simulink model "Inverter2016a"  (R2016a)
settings: Solver=VariableStepAuto  SolverMode=SingleTasking  StartTime=0.0  StopTime=30e-3  FixedStep=SampleTime  MinStep=SampleTime*1e-2  RelTol=1e-3
values from neighbouring files (symbols this model uses):
  ffund = 50    [InverterMFile.m]
  ModulationIndex = 0.9    [InverterMFile.m]
  Rin = 10    [InverterMFile.m]
  Rload = Z*PF    [InverterMFile.m]
  VpulseMax = 6    [InverterMFile.m]
  VpulseMin = -3    [InverterMFile.m]
libraries: elec_lib x135, fl_lib x66, nesl_utility x65, simulink x24, powerlib_meascontrol x2
(part 4 of 4)

== system Inverter2016a/3ph- Module1/Gate Driver5 ==
  PWM : Inport
  Capacitor : elec_lib/Passive Devices/Capacitor  enable_table=0  c=142e-12 F  Cvec=[1e-05, 1e-06] F  Vvec=[0, 10] V  CV_table_symmetry=1  C_tol=5  enable_C_tol=0  tol_distribution=1  nSigma=4  r=1e-6 Ohm  g=0 1/Ohm  enable_operating_limits=0  operating_limit_action=2  max_working_voltage_range=[-25, 25] V  power_rating=1 W  enable_faults=0  fault_action=1  Cscale_faulted=100  R_faulted=1e-3 Ohm  G_faulted=0 1/Ohm  tau_fault=1e-3 s  enable_temporal_fault=0  t_fault=1 s  enable_behavioral_fault=0  max_permissible_voltage_range=[-100, 100] V  t_fail_on_voltage=1 s  i_specify=off  i_priority=None  i=0 A  i_nominal_specify=off  i_nominal_unit=A  i_nominal_value=1  v_specify=off  v_priority=None  v=0 V  v_nominal_specify=off  v_nominal_unit=V  v_nominal_value=1  vc_specify=off  vc_priority=High  vc=0 V  vc_nominal_specify=off  vc_nominal_unit=V  vc_nominal_value=1
  Current Measure : Subsystem
  Inductor : elec_lib/Passive Devices/Inductor  l=Ls H  L_tol=20  enable_L_tol=0  tol_distribution=1  nSigma=4  r=0 Ohm  g=1e-9 1/Ohm  enable_operating_limits=0  operating_limit_action=2  max_working_current=1 A  power_rating=1 W  enable_faults=0  fault_action=1  lambdaPercent=50  k_faulted=0.9999  turnsShort=0  openCct=0  groundShort=0  groundShortG=0 1/Ohm  tau_fault=1e-3 s  enable_temporal_fault=0  t_fault=1 s  enable_behavioral_fault=0  max_permissible_voltage=100 V  n_fail_on_voltage=1  max_permissible_current=1 A  t_fail_on_current=1 s  i_L_specify=off  i_L_priority=High  i_L=0 A  i_L_nominal_specify=off  i_L_nominal_unit=A  i_L_nominal_value=1
  Inductor1 : elec_lib/Passive Devices/Inductor  l=Ld H  L_tol=20  enable_L_tol=0  tol_distribution=1  nSigma=4  r=0 Ohm  g=1e-9 1/Ohm  enable_operating_limits=0  operating_limit_action=2  max_working_current=1 A  power_rating=1 W  enable_faults=0  fault_action=1  lambdaPercent=50  k_faulted=0.9999  turnsShort=0  openCct=0  groundShort=0  groundShortG=0 1/Ohm  tau_fault=1e-3 s  enable_temporal_fault=0  t_fault=1 s  enable_behavioral_fault=0  max_permissible_voltage=100 V  n_fail_on_voltage=1  max_permissible_current=1 A  t_fail_on_current=1 s  i_L_specify=off  i_L_priority=High  i_L=0 A  i_L_nominal_specify=off  i_L_nominal_unit=A  i_L_nominal_value=1
  Rate Limiter2 : Subsystem
  Simulink-PS Converter : nesl_utility/Simulink-PS Converter  PhysicalDomain=network_engine_domain  SubClassName=ps_input  LeftPortType=input  RightPortType=output  PseudoPeriodic=off  Frequencies=[]  NoiseDistribution=none  NoiseParameters=[]  Unit=1  AffineConversion=off  FilteringAndDerivatives=zero  SimscapeFilterOrder=1  InputFilterTimeConstant=0.001  UdotUserProvided=1
  Switch6 : fl_lib/Electrical/Electrical Elements/Switch  R_closed=0.05 Ohm  G_open=1e-8 1/Ohm  Threshold=1.7  i_specify=off  i_priority=None  i=0 A  i_nominal_specify=off  i_nominal_unit=A  i_nominal_value=1  v_specify=off  v_priority=None  v=0 V  v_nominal_specify=off  v_nominal_unit=V  v_nominal_value=1
  Voltage Measure3 : Subsystem
  Drain : PMIOPort  Side=Left
  Source : PMIOPort  Port=2  Side=Right
  Volt : Outport
  Curr : Outport  Port=2
  wires:
  Current Measure/1(Data) -> Curr/1
  Voltage Measure3/1(Data) -> Volt/1
  Rate Limiter2/1(Outp) -> Simulink-PS Converter/1
  PWM/1 -> Rate Limiter2/1(Inp)
  connections:
  Current Measure/RConn1 -- Inductor1/RConn1
  Inductor/RConn1 -- Source/RConn1
  Current Measure/LConn1 -- Drain/RConn1
  Inductor1/LConn1 -- Capacitor/LConn1 -- Switch6/LConn1 -- Voltage Measure3/RConn1
  Capacitor/RConn1 -- Voltage Measure3/RConn2 -- Switch6/RConn2 -- Inductor/LConn1
  Switch6/RConn1 -- Simulink-PS Converter/RConn1

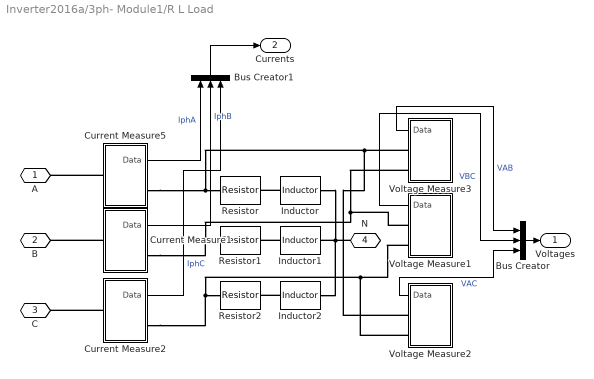
== system Inverter2016a/3ph- Module1/R L Load ==
  Bus Creator : BusCreator  Inputs=3
  Bus Creator1 : BusCreator  Inputs=3
  Current Measure1 : Subsystem
  Current Measure2 : Subsystem
  Current Measure5 : Subsystem
  Inductor : elec_lib/Passive Devices/Inductor  l=Lload H  L_tol=20  enable_L_tol=0  tol_distribution=1  nSigma=4  r=0 Ohm  g=1e-9 1/Ohm  enable_operating_limits=0  operating_limit_action=2  max_working_current=1 A  power_rating=1 W  enable_faults=0  fault_action=1  lambdaPercent=50  k_faulted=0.9999  turnsShort=0  openCct=0  groundShort=0  groundShortG=0 1/Ohm  tau_fault=0.001 s  enable_temporal_fault=0  t_fault=1 s  enable_behavioral_fault=0  max_permissible_voltage=100 V  n_fail_on_voltage=1  max_permissible_current=1 A  t_fail_on_current=1 s  i_L_specify=on  i_L_priority=High  i_L=LoadA A  i_L_nominal_specify=off  i_L_nominal_unit=A  i_L_nominal_value=1
  Inductor1 : elec_lib/Passive Devices/Inductor  l=Lload H  L_tol=20  enable_L_tol=0  tol_distribution=1  nSigma=4  r=0 Ohm  g=1e-9 1/Ohm  enable_operating_limits=0  operating_limit_action=2  max_working_current=1 A  power_rating=1 W  enable_faults=0  fault_action=1  lambdaPercent=50  k_faulted=0.9999  turnsShort=0  openCct=0  groundShort=0  groundShortG=0 1/Ohm  tau_fault=0.001 s  enable_temporal_fault=0  t_fault=1 s  enable_behavioral_fault=0  max_permissible_voltage=100 V  n_fail_on_voltage=1  max_permissible_current=1 A  t_fail_on_current=1 s  i_L_specify=on  i_L_priority=High  i_L=LoadB A  i_L_nominal_specify=off  i_L_nominal_unit=A  i_L_nominal_value=1
  Inductor2 : elec_lib/Passive Devices/Inductor  l=Lload H  L_tol=20  enable_L_tol=0  tol_distribution=1  nSigma=4  r=0 Ohm  g=1e-9 1/Ohm  enable_operating_limits=0  operating_limit_action=2  max_working_current=1 A  power_rating=1 W  enable_faults=0  fault_action=1  lambdaPercent=50  k_faulted=0.9999  turnsShort=0  openCct=0  groundShort=0  groundShortG=0 1/Ohm  tau_fault=0.001 s  enable_temporal_fault=0  t_fault=1 s  enable_behavioral_fault=0  max_permissible_voltage=100 V  n_fail_on_voltage=1  max_permissible_current=1 A  t_fail_on_current=1 s  i_L_specify=on  i_L_priority=High  i_L=LoadC A  i_L_nominal_specify=off  i_L_nominal_unit=A  i_L_nominal_value=1
  Resistor : elec_lib/Passive Devices/Resistor  R=Rload Ohm  R_tol=5  enable_R_tol=0  tol_distribution=1  nSigma=4  enable_operating_limits=0  operating_limit_action=2  max_working_voltage=100 V  power_rating=1 W  enable_faults=0  fault_action=1  R_faulted=Inf Ohm  enable_temporal_fault=0  t_fault=1 s  enable_behavioral_fault=0  max_permissible_current=1 A  t_fail_on_current=1 s  noise_mode=0  sample_time=0.001 s  repeatability=1  auto_seed=851356125  user_seed=0  Tdevice=25 degC  alpha=3.93e-3 1/K  Tmeas=25 degC  thermal_mass=100 J/K  power_derating_T1=70 degC  power_derating_T2=155 degC  operating_temperature_range_vec=[-50, 150] degC  temperature_specify=off  temperature_priority=High  temperature=298.15 K  temperature_nominal_specify=off  temperature_nominal_unit=K  temperature_nominal_value=1
  Resistor1 : elec_lib/Passive Devices/Resistor  R=Rload Ohm  R_tol=5  enable_R_tol=0  tol_distribution=1  nSigma=4  enable_operating_limits=0  operating_limit_action=2  max_working_voltage=100 V  power_rating=1 W  enable_faults=0  fault_action=1  R_faulted=Inf Ohm  enable_temporal_fault=0  t_fault=1 s  enable_behavioral_fault=0  max_permissible_current=1 A  t_fail_on_current=1 s  noise_mode=0  sample_time=0.001 s  repeatability=1  auto_seed=837825856  user_seed=0  Tdevice=25 degC  alpha=3.93e-3 1/K  Tmeas=25 degC  thermal_mass=100 J/K  power_derating_T1=70 degC  power_derating_T2=155 degC  operating_temperature_range_vec=[-50, 150] degC  temperature_specify=off  temperature_priority=High  temperature=298.15 K  temperature_nominal_specify=off  temperature_nominal_unit=K  temperature_nominal_value=1
  Resistor2 : elec_lib/Passive Devices/Resistor  R=Rload Ohm  R_tol=5  enable_R_tol=0  tol_distribution=1  nSigma=4  enable_operating_limits=0  operating_limit_action=2  max_working_voltage=100 V  power_rating=1 W  enable_faults=0  fault_action=1  R_faulted=Inf Ohm  enable_temporal_fault=0  t_fault=1 s  enable_behavioral_fault=0  max_permissible_current=1 A  t_fail_on_current=1 s  noise_mode=0  sample_time=0.001 s  repeatability=1  auto_seed=1403765601  user_seed=0  Tdevice=25 degC  alpha=3.93e-3 1/K  Tmeas=25 degC  thermal_mass=100 J/K  power_derating_T1=70 degC  power_derating_T2=155 degC  operating_temperature_range_vec=[-50, 150] degC  temperature_specify=off  temperature_priority=High  temperature=298.15 K  temperature_nominal_specify=off  temperature_nominal_unit=K  temperature_nominal_value=1
  Voltage Measure1 : Subsystem
  Voltage Measure2 : Subsystem
  Voltage Measure3 : Subsystem
  A : PMIOPort  Side=Left
  B : PMIOPort  Port=2  Side=Left
  C : PMIOPort  Port=3  Side=Left
  N : PMIOPort  Port=4  Side=Right
  Voltages : Outport
  Currents : Outport  Port=2
  wires:
  Bus Creator1/1 -> Currents/1
  Bus Creator/1 -> Voltages/1
  Current Measure2/1(Data) -> Bus Creator1/3  "IphC"
  Current Measure1/1(Data) -> Bus Creator1/2  "IphB"
  Current Measure5/1(Data) -> Bus Creator1/1  "IphA"
  Voltage Measure2/1(Data) -> Bus Creator/3  "VAC"
  Voltage Measure1/1(Data) -> Bus Creator/2  "VBC"
  Voltage Measure3/1(Data) -> Bus Creator/1  "VAB"
  connections:
  Current Measure2/LConn1 -- C/RConn1
  Current Measure1/LConn1 -- B/RConn1
  Current Measure5/LConn1 -- A/RConn1
  Resistor2/LConn1 -- Voltage Measure1/RConn2 -- Voltage Measure2/RConn2 -- Current Measure2/RConn1
  Resistor/LConn1 -- Voltage Measure3/RConn1 -- Voltage Measure2/RConn1 -- Current Measure5/RConn1
  Resistor1/LConn1 -- Voltage Measure3/RConn2 -- Voltage Measure1/RConn1 -- Current Measure1/RConn1
  Inductor1/LConn1 -- Resistor1/RConn1
  Inductor2/LConn1 -- Resistor2/RConn1
  N/RConn1 -- Inductor1/RConn1 -- Inductor2/RConn1 -- Inductor/RConn1
  Inductor/LConn1 -- Resistor/RConn1

== system Inverter2016a/3ph- Module1/Voltage Measure1 ==
  PS-Simulink Converter2 : nesl_utility/PS-Simulink Converter  PhysicalDomain=network_engine_domain  SubClassName=ps_output  LeftPortType=input  RightPortType=output  PseudoPeriodic=off  Frequencies=[]  Unit=1  AffineConversion=off
  Voltage Sensor3 : fl_lib/Electrical/Electrical Sensors/Voltage Sensor
  V+ : PMIOPort  Side=Right
  V- : PMIOPort  Port=2  Side=Right
  Data : Outport
  wires:
  PS-Simulink Converter2/1 -> Data/1
  connections:
  PS-Simulink Converter2/LConn1 -- Voltage Sensor3/RConn1
  Voltage Sensor3/RConn2 -- V-/RConn1
  Voltage Sensor3/LConn1 -- V+/RConn1

== system Inverter2016a/3ph- Module1/Voltage Measure2 ==
  PS-Simulink Converter2 : nesl_utility/PS-Simulink Converter  PhysicalDomain=network_engine_domain  SubClassName=ps_output  LeftPortType=input  RightPortType=output  PseudoPeriodic=off  Frequencies=[]  Unit=1  AffineConversion=off
  Voltage Sensor3 : fl_lib/Electrical/Electrical Sensors/Voltage Sensor
  V+ : PMIOPort  Side=Right
  V- : PMIOPort  Port=2  Side=Right
  Data : Outport
  wires:
  PS-Simulink Converter2/1 -> Data/1
  connections:
  PS-Simulink Converter2/LConn1 -- Voltage Sensor3/RConn1
  Voltage Sensor3/RConn2 -- V-/RConn1
  Voltage Sensor3/LConn1 -- V+/RConn1

== system Inverter2016a/3ph- Module1/Voltage Measure3 ==
  PS-Simulink Converter2 : nesl_utility/PS-Simulink Converter  PhysicalDomain=network_engine_domain  SubClassName=ps_output  LeftPortType=input  RightPortType=output  PseudoPeriodic=off  Frequencies=[]  Unit=1  AffineConversion=off
  Voltage Sensor3 : fl_lib/Electrical/Electrical Sensors/Voltage Sensor
  V+ : PMIOPort  Side=Right
  V- : PMIOPort  Port=2  Side=Right
  Data : Outport
  wires:
  PS-Simulink Converter2/1 -> Data/1
  connections:
  PS-Simulink Converter2/LConn1 -- Voltage Sensor3/RConn1
  Voltage Sensor3/RConn2 -- V-/RConn1
  Voltage Sensor3/LConn1 -- V+/RConn1

== system Inverter2016a/3ph- Module1/Voltage Measure4 ==
  PS-Simulink Converter2 : nesl_utility/PS-Simulink Converter  PhysicalDomain=network_engine_domain  SubClassName=ps_output  LeftPortType=input  RightPortType=output  PseudoPeriodic=off  Frequencies=[]  Unit=1  AffineConversion=off
  Voltage Sensor3 : fl_lib/Electrical/Electrical Sensors/Voltage Sensor
  V+ : PMIOPort  Side=Right
  V- : PMIOPort  Port=2  Side=Right
  Data : Outport
  wires:
  PS-Simulink Converter2/1 -> Data/1
  connections:
  Voltage Sensor3/LConn1 -- V+/RConn1
  Voltage Sensor3/RConn2 -- V-/RConn1
  PS-Simulink Converter2/LConn1 -- Voltage Sensor3/RConn1

== system Inverter2016a/3ph- Module/Gate Driver/Current Measure ==
  Current Sensor1 : fl_lib/Electrical/Electrical Sensors/Current Sensor
  PS-Simulink Converter4 : nesl_utility/PS-Simulink Converter  PhysicalDomain=network_engine_domain  SubClassName=ps_output  LeftPortType=input  RightPortType=output  PseudoPeriodic=off  Frequencies=[]  Unit=1  AffineConversion=off
  I+ : PMIOPort  Side=Left
  I- : PMIOPort  Port=2  Side=Right
  Data : Outport
  wires:
  PS-Simulink Converter4/1 -> Data/1
  connections:
  Current Sensor1/RConn2 -- I-/RConn1
  PS-Simulink Converter4/LConn1 -- Current Sensor1/RConn1
  Current Sensor1/LConn1 -- I+/RConn1

== system Inverter2016a/3ph- Module/Gate Driver/Rate Limiter2 ==
  Inp : Inport
  Constant2 : Constant  Value=(VpulseMax - VpulseMin)/1e-9
  Constant3 : Constant  Value=(VpulseMin - VpulseMax)/1e-9
  Rate Limiter Dynamic : simulink/Discontinuities/Rate Limiter Dynamic
  Outp : Outport
  wires:
  Constant3/1 -> Rate Limiter Dynamic/3
  Constant2/1 -> Rate Limiter Dynamic/1
  Inp/1 -> Rate Limiter Dynamic/2
  Rate Limiter Dynamic/1 -> Outp/1

== system Inverter2016a/3ph- Module/Gate Driver/Voltage Measure3 ==
  PS-Simulink Converter2 : nesl_utility/PS-Simulink Converter  PhysicalDomain=network_engine_domain  SubClassName=ps_output  LeftPortType=input  RightPortType=output  PseudoPeriodic=off  Frequencies=[]  Unit=1  AffineConversion=off
  Voltage Sensor3 : fl_lib/Electrical/Electrical Sensors/Voltage Sensor
  V+ : PMIOPort  Side=Right
  V- : PMIOPort  Port=2  Side=Right
  Data : Outport
  wires:
  PS-Simulink Converter2/1 -> Data/1
  connections:
  Voltage Sensor3/LConn1 -- V+/RConn1
  Voltage Sensor3/RConn2 -- V-/RConn1
  PS-Simulink Converter2/LConn1 -- Voltage Sensor3/RConn1

== system Inverter2016a/3ph- Module/Gate Driver1/Current Measure ==
  Current Sensor1 : fl_lib/Electrical/Electrical Sensors/Current Sensor
  PS-Simulink Converter4 : nesl_utility/PS-Simulink Converter  PhysicalDomain=network_engine_domain  SubClassName=ps_output  LeftPortType=input  RightPortType=output  PseudoPeriodic=off  Frequencies=[]  Unit=1  AffineConversion=off
  I+ : PMIOPort  Side=Left
  I- : PMIOPort  Port=2  Side=Right
  Data : Outport
  wires:
  PS-Simulink Converter4/1 -> Data/1
  connections:
  Current Sensor1/RConn2 -- I-/RConn1
  PS-Simulink Converter4/LConn1 -- Current Sensor1/RConn1
  Current Sensor1/LConn1 -- I+/RConn1

== system Inverter2016a/3ph- Module/Gate Driver1/Rate Limiter2 ==
  Inp : Inport
  Constant2 : Constant  Value=(VpulseMax - VpulseMin)/1e-9
  Constant3 : Constant  Value=(VpulseMin - VpulseMax)/1e-9
  Rate Limiter Dynamic : simulink/Discontinuities/Rate Limiter Dynamic
  Outp : Outport
  wires:
  Constant3/1 -> Rate Limiter Dynamic/3
  Constant2/1 -> Rate Limiter Dynamic/1
  Inp/1 -> Rate Limiter Dynamic/2
  Rate Limiter Dynamic/1 -> Outp/1

== system Inverter2016a/3ph- Module/Gate Driver1/Voltage Measure3 ==
  PS-Simulink Converter2 : nesl_utility/PS-Simulink Converter  PhysicalDomain=network_engine_domain  SubClassName=ps_output  LeftPortType=input  RightPortType=output  PseudoPeriodic=off  Frequencies=[]  Unit=1  AffineConversion=off
  Voltage Sensor3 : fl_lib/Electrical/Electrical Sensors/Voltage Sensor
  V+ : PMIOPort  Side=Right
  V- : PMIOPort  Port=2  Side=Right
  Data : Outport
  wires:
  PS-Simulink Converter2/1 -> Data/1
  connections:
  Voltage Sensor3/LConn1 -- V+/RConn1
  Voltage Sensor3/RConn2 -- V-/RConn1
  PS-Simulink Converter2/LConn1 -- Voltage Sensor3/RConn1

== system Inverter2016a/3ph- Module/Gate Driver2/Current Measure ==
  Current Sensor1 : fl_lib/Electrical/Electrical Sensors/Current Sensor
  PS-Simulink Converter4 : nesl_utility/PS-Simulink Converter  PhysicalDomain=network_engine_domain  SubClassName=ps_output  LeftPortType=input  RightPortType=output  PseudoPeriodic=off  Frequencies=[]  Unit=1  AffineConversion=off
  I+ : PMIOPort  Side=Left
  I- : PMIOPort  Port=2  Side=Right
  Data : Outport
  wires:
  PS-Simulink Converter4/1 -> Data/1
  connections:
  Current Sensor1/RConn2 -- I-/RConn1
  PS-Simulink Converter4/LConn1 -- Current Sensor1/RConn1
  Current Sensor1/LConn1 -- I+/RConn1

== system Inverter2016a/3ph- Module/Gate Driver2/Rate Limiter2 ==
  Inp : Inport
  Constant2 : Constant  Value=(VpulseMax - VpulseMin)/1e-9
  Constant3 : Constant  Value=(VpulseMin - VpulseMax)/1e-9
  Rate Limiter Dynamic : simulink/Discontinuities/Rate Limiter Dynamic
  Outp : Outport
  wires:
  Constant3/1 -> Rate Limiter Dynamic/3
  Constant2/1 -> Rate Limiter Dynamic/1
  Inp/1 -> Rate Limiter Dynamic/2
  Rate Limiter Dynamic/1 -> Outp/1

== system Inverter2016a/3ph- Module/Gate Driver2/Voltage Measure3 ==
  PS-Simulink Converter2 : nesl_utility/PS-Simulink Converter  PhysicalDomain=network_engine_domain  SubClassName=ps_output  LeftPortType=input  RightPortType=output  PseudoPeriodic=off  Frequencies=[]  Unit=1  AffineConversion=off
  Voltage Sensor3 : fl_lib/Electrical/Electrical Sensors/Voltage Sensor
  V+ : PMIOPort  Side=Right
  V- : PMIOPort  Port=2  Side=Right
  Data : Outport
  wires:
  PS-Simulink Converter2/1 -> Data/1
  connections:
  Voltage Sensor3/LConn1 -- V+/RConn1
  Voltage Sensor3/RConn2 -- V-/RConn1
  PS-Simulink Converter2/LConn1 -- Voltage Sensor3/RConn1

== system Inverter2016a/3ph- Module/Gate Driver3/Current Measure ==
  Current Sensor1 : fl_lib/Electrical/Electrical Sensors/Current Sensor
  PS-Simulink Converter4 : nesl_utility/PS-Simulink Converter  PhysicalDomain=network_engine_domain  SubClassName=ps_output  LeftPortType=input  RightPortType=output  PseudoPeriodic=off  Frequencies=[]  Unit=1  AffineConversion=off
  I+ : PMIOPort  Side=Left
  I- : PMIOPort  Port=2  Side=Right
  Data : Outport
  wires:
  PS-Simulink Converter4/1 -> Data/1
  connections:
  Current Sensor1/RConn2 -- I-/RConn1
  PS-Simulink Converter4/LConn1 -- Current Sensor1/RConn1
  Current Sensor1/LConn1 -- I+/RConn1

== system Inverter2016a/3ph- Module/Gate Driver3/Rate Limiter2 ==
  Inp : Inport
  Constant2 : Constant  Value=(VpulseMax - VpulseMin)/1e-9
  Constant3 : Constant  Value=(VpulseMin - VpulseMax)/1e-9
  Rate Limiter Dynamic : simulink/Discontinuities/Rate Limiter Dynamic
  Outp : Outport
  wires:
  Constant3/1 -> Rate Limiter Dynamic/3
  Constant2/1 -> Rate Limiter Dynamic/1
  Inp/1 -> Rate Limiter Dynamic/2
  Rate Limiter Dynamic/1 -> Outp/1

== system Inverter2016a/3ph- Module/Gate Driver3/Voltage Measure3 ==
  PS-Simulink Converter2 : nesl_utility/PS-Simulink Converter  PhysicalDomain=network_engine_domain  SubClassName=ps_output  LeftPortType=input  RightPortType=output  PseudoPeriodic=off  Frequencies=[]  Unit=1  AffineConversion=off
  Voltage Sensor3 : fl_lib/Electrical/Electrical Sensors/Voltage Sensor
  V+ : PMIOPort  Side=Right
  V- : PMIOPort  Port=2  Side=Right
  Data : Outport
  wires:
  PS-Simulink Converter2/1 -> Data/1
  connections:
  Voltage Sensor3/LConn1 -- V+/RConn1
  Voltage Sensor3/RConn2 -- V-/RConn1
  PS-Simulink Converter2/LConn1 -- Voltage Sensor3/RConn1

== system Inverter2016a/3ph- Module/Gate Driver4/Current Measure ==
  Current Sensor1 : fl_lib/Electrical/Electrical Sensors/Current Sensor
  PS-Simulink Converter4 : nesl_utility/PS-Simulink Converter  PhysicalDomain=network_engine_domain  SubClassName=ps_output  LeftPortType=input  RightPortType=output  PseudoPeriodic=off  Frequencies=[]  Unit=1  AffineConversion=off
  I+ : PMIOPort  Side=Left
  I- : PMIOPort  Port=2  Side=Right
  Data : Outport
  wires:
  PS-Simulink Converter4/1 -> Data/1
  connections:
  Current Sensor1/RConn2 -- I-/RConn1
  PS-Simulink Converter4/LConn1 -- Current Sensor1/RConn1
  Current Sensor1/LConn1 -- I+/RConn1

== system Inverter2016a/3ph- Module/Gate Driver4/Rate Limiter2 ==
  Inp : Inport
  Constant2 : Constant  Value=(VpulseMax - VpulseMin)/1e-9
  Constant3 : Constant  Value=(VpulseMin - VpulseMax)/1e-9
  Rate Limiter Dynamic : simulink/Discontinuities/Rate Limiter Dynamic
  Outp : Outport
  wires:
  Constant3/1 -> Rate Limiter Dynamic/3
  Constant2/1 -> Rate Limiter Dynamic/1
  Inp/1 -> Rate Limiter Dynamic/2
  Rate Limiter Dynamic/1 -> Outp/1

== system Inverter2016a/3ph- Module/Gate Driver4/Voltage Measure3 ==
  PS-Simulink Converter2 : nesl_utility/PS-Simulink Converter  PhysicalDomain=network_engine_domain  SubClassName=ps_output  LeftPortType=input  RightPortType=output  PseudoPeriodic=off  Frequencies=[]  Unit=1  AffineConversion=off
  Voltage Sensor3 : fl_lib/Electrical/Electrical Sensors/Voltage Sensor
  V+ : PMIOPort  Side=Right
  V- : PMIOPort  Port=2  Side=Right
  Data : Outport
  wires:
  PS-Simulink Converter2/1 -> Data/1
  connections:
  Voltage Sensor3/LConn1 -- V+/RConn1
  Voltage Sensor3/RConn2 -- V-/RConn1
  PS-Simulink Converter2/LConn1 -- Voltage Sensor3/RConn1

== system Inverter2016a/3ph- Module/Gate Driver5/Current Measure ==
  Current Sensor1 : fl_lib/Electrical/Electrical Sensors/Current Sensor
  PS-Simulink Converter4 : nesl_utility/PS-Simulink Converter  PhysicalDomain=network_engine_domain  SubClassName=ps_output  LeftPortType=input  RightPortType=output  PseudoPeriodic=off  Frequencies=[]  Unit=1  AffineConversion=off
  I+ : PMIOPort  Side=Left
  I- : PMIOPort  Port=2  Side=Right
  Data : Outport
  wires:
  PS-Simulink Converter4/1 -> Data/1
  connections:
  Current Sensor1/RConn2 -- I-/RConn1
  PS-Simulink Converter4/LConn1 -- Current Sensor1/RConn1
  Current Sensor1/LConn1 -- I+/RConn1

== system Inverter2016a/3ph- Module/Gate Driver5/Rate Limiter2 ==
  Inp : Inport
  Constant2 : Constant  Value=(VpulseMax - VpulseMin)/1e-9
  Constant3 : Constant  Value=(VpulseMin - VpulseMax)/1e-9
  Rate Limiter Dynamic : simulink/Discontinuities/Rate Limiter Dynamic
  Outp : Outport
  wires:
  Constant3/1 -> Rate Limiter Dynamic/3
  Constant2/1 -> Rate Limiter Dynamic/1
  Inp/1 -> Rate Limiter Dynamic/2
  Rate Limiter Dynamic/1 -> Outp/1

== system Inverter2016a/3ph- Module/Gate Driver5/Voltage Measure3 ==
  PS-Simulink Converter2 : nesl_utility/PS-Simulink Converter  PhysicalDomain=network_engine_domain  SubClassName=ps_output  LeftPortType=input  RightPortType=output  PseudoPeriodic=off  Frequencies=[]  Unit=1  AffineConversion=off
  Voltage Sensor3 : fl_lib/Electrical/Electrical Sensors/Voltage Sensor
  V+ : PMIOPort  Side=Right
  V- : PMIOPort  Port=2  Side=Right
  Data : Outport
  wires:
  PS-Simulink Converter2/1 -> Data/1
  connections:
  Voltage Sensor3/LConn1 -- V+/RConn1
  Voltage Sensor3/RConn2 -- V-/RConn1
  PS-Simulink Converter2/LConn1 -- Voltage Sensor3/RConn1

== system Inverter2016a/3ph- Module/R L Load/Current Measure1 ==
  Current Sensor1 : fl_lib/Electrical/Electrical Sensors/Current Sensor
  PS-Simulink Converter4 : nesl_utility/PS-Simulink Converter  PhysicalDomain=network_engine_domain  SubClassName=ps_output  LeftPortType=input  RightPortType=output  PseudoPeriodic=off  Frequencies=[]  Unit=1  AffineConversion=off
  I+ : PMIOPort  Side=Left
  I- : PMIOPort  Port=2  Side=Right
  Data : Outport
  wires:
  PS-Simulink Converter4/1 -> Data/1
  connections:
  Current Sensor1/LConn1 -- I+/RConn1
  PS-Simulink Converter4/LConn1 -- Current Sensor1/RConn1
  Current Sensor1/RConn2 -- I-/RConn1

== system Inverter2016a/3ph- Module/R L Load/Current Measure2 ==
  Current Sensor1 : fl_lib/Electrical/Electrical Sensors/Current Sensor
  PS-Simulink Converter4 : nesl_utility/PS-Simulink Converter  PhysicalDomain=network_engine_domain  SubClassName=ps_output  LeftPortType=input  RightPortType=output  PseudoPeriodic=off  Frequencies=[]  Unit=1  AffineConversion=off
  I+ : PMIOPort  Side=Left
  I- : PMIOPort  Port=2  Side=Right
  Data : Outport
  wires:
  PS-Simulink Converter4/1 -> Data/1
  connections:
  Current Sensor1/RConn2 -- I-/RConn1
  PS-Simulink Converter4/LConn1 -- Current Sensor1/RConn1
  Current Sensor1/LConn1 -- I+/RConn1

== system Inverter2016a/3ph- Module/R L Load/Current Measure5 ==
  Current Sensor1 : fl_lib/Electrical/Electrical Sensors/Current Sensor
  PS-Simulink Converter4 : nesl_utility/PS-Simulink Converter  PhysicalDomain=network_engine_domain  SubClassName=ps_output  LeftPortType=input  RightPortType=output  PseudoPeriodic=off  Frequencies=[]  Unit=1  AffineConversion=off
  I+ : PMIOPort  Side=Left
  I- : PMIOPort  Port=2  Side=Right
  Data : Outport
  wires:
  PS-Simulink Converter4/1 -> Data/1
  connections:
  Current Sensor1/RConn2 -- I-/RConn1
  PS-Simulink Converter4/LConn1 -- Current Sensor1/RConn1
  Current Sensor1/LConn1 -- I+/RConn1

== system Inverter2016a/3ph- Module/R L Load/Voltage Measure1 ==
  PS-Simulink Converter2 : nesl_utility/PS-Simulink Converter  PhysicalDomain=network_engine_domain  SubClassName=ps_output  LeftPortType=input  RightPortType=output  PseudoPeriodic=off  Frequencies=[]  Unit=1  AffineConversion=off
  Voltage Sensor3 : fl_lib/Electrical/Electrical Sensors/Voltage Sensor
  V+ : PMIOPort  Side=Right
  V- : PMIOPort  Port=2  Side=Right
  Data : Outport
  wires:
  PS-Simulink Converter2/1 -> Data/1
  connections:
  PS-Simulink Converter2/LConn1 -- Voltage Sensor3/RConn1
  Voltage Sensor3/RConn2 -- V-/RConn1
  Voltage Sensor3/LConn1 -- V+/RConn1

== system Inverter2016a/3ph- Module/R L Load/Voltage Measure2 ==
  PS-Simulink Converter2 : nesl_utility/PS-Simulink Converter  PhysicalDomain=network_engine_domain  SubClassName=ps_output  LeftPortType=input  RightPortType=output  PseudoPeriodic=off  Frequencies=[]  Unit=1  AffineConversion=off
  Voltage Sensor3 : fl_lib/Electrical/Electrical Sensors/Voltage Sensor
  V+ : PMIOPort  Side=Right
  V- : PMIOPort  Port=2  Side=Right
  Data : Outport
  wires:
  PS-Simulink Converter2/1 -> Data/1
  connections:
  Voltage Sensor3/LConn1 -- V+/RConn1
  Voltage Sensor3/RConn2 -- V-/RConn1
  PS-Simulink Converter2/LConn1 -- Voltage Sensor3/RConn1

== system Inverter2016a/3ph- Module/R L Load/Voltage Measure3 ==
  PS-Simulink Converter2 : nesl_utility/PS-Simulink Converter  PhysicalDomain=network_engine_domain  SubClassName=ps_output  LeftPortType=input  RightPortType=output  PseudoPeriodic=off  Frequencies=[]  Unit=1  AffineConversion=off
  Voltage Sensor3 : fl_lib/Electrical/Electrical Sensors/Voltage Sensor
  V+ : PMIOPort  Side=Right
  V- : PMIOPort  Port=2  Side=Right
  Data : Outport
  wires:
  PS-Simulink Converter2/1 -> Data/1
  connections:
  Voltage Sensor3/LConn1 -- V+/RConn1
  Voltage Sensor3/RConn2 -- V-/RConn1
  PS-Simulink Converter2/LConn1 -- Voltage Sensor3/RConn1

== system Inverter2016a/3ph- Module1/Gate Driver/Current Measure ==
  Current Sensor1 : fl_lib/Electrical/Electrical Sensors/Current Sensor
  PS-Simulink Converter4 : nesl_utility/PS-Simulink Converter  PhysicalDomain=network_engine_domain  SubClassName=ps_output  LeftPortType=input  RightPortType=output  PseudoPeriodic=off  Frequencies=[]  Unit=1  AffineConversion=off
  I+ : PMIOPort  Side=Left
  I- : PMIOPort  Port=2  Side=Right
  Data : Outport
  wires:
  PS-Simulink Converter4/1 -> Data/1
  connections:
  Current Sensor1/LConn1 -- I+/RConn1
  PS-Simulink Converter4/LConn1 -- Current Sensor1/RConn1
  Current Sensor1/RConn2 -- I-/RConn1

== system Inverter2016a/3ph- Module1/Gate Driver/Rate Limiter2 ==
  Inp : Inport
  Constant2 : Constant  Value=(VpulseMax - VpulseMin)/1e-9
  Constant3 : Constant  Value=(VpulseMin - VpulseMax)/1e-9
  Rate Limiter Dynamic : simulink/Discontinuities/Rate Limiter Dynamic
  Outp : Outport
  wires:
  Rate Limiter Dynamic/1 -> Outp/1
  Inp/1 -> Rate Limiter Dynamic/2
  Constant2/1 -> Rate Limiter Dynamic/1
  Constant3/1 -> Rate Limiter Dynamic/3

== system Inverter2016a/3ph- Module1/Gate Driver/Voltage Measure3 ==
  PS-Simulink Converter2 : nesl_utility/PS-Simulink Converter  PhysicalDomain=network_engine_domain  SubClassName=ps_output  LeftPortType=input  RightPortType=output  PseudoPeriodic=off  Frequencies=[]  Unit=1  AffineConversion=off
  Voltage Sensor3 : fl_lib/Electrical/Electrical Sensors/Voltage Sensor
  V+ : PMIOPort  Side=Right
  V- : PMIOPort  Port=2  Side=Right
  Data : Outport
  wires:
  PS-Simulink Converter2/1 -> Data/1
  connections:
  PS-Simulink Converter2/LConn1 -- Voltage Sensor3/RConn1
  Voltage Sensor3/RConn2 -- V-/RConn1
  Voltage Sensor3/LConn1 -- V+/RConn1

== system Inverter2016a/3ph- Module1/Gate Driver1/Current Measure ==
  Current Sensor1 : fl_lib/Electrical/Electrical Sensors/Current Sensor
  PS-Simulink Converter4 : nesl_utility/PS-Simulink Converter  PhysicalDomain=network_engine_domain  SubClassName=ps_output  LeftPortType=input  RightPortType=output  PseudoPeriodic=off  Frequencies=[]  Unit=1  AffineConversion=off
  I+ : PMIOPort  Side=Left
  I- : PMIOPort  Port=2  Side=Right
  Data : Outport
  wires:
  PS-Simulink Converter4/1 -> Data/1
  connections:
  Current Sensor1/LConn1 -- I+/RConn1
  PS-Simulink Converter4/LConn1 -- Current Sensor1/RConn1
  Current Sensor1/RConn2 -- I-/RConn1

== system Inverter2016a/3ph- Module1/Gate Driver1/Rate Limiter2 ==
  Inp : Inport
  Constant2 : Constant  Value=(VpulseMax - VpulseMin)/1e-9
  Constant3 : Constant  Value=(VpulseMin - VpulseMax)/1e-9
  Rate Limiter Dynamic : simulink/Discontinuities/Rate Limiter Dynamic
  Outp : Outport
  wires:
  Rate Limiter Dynamic/1 -> Outp/1
  Inp/1 -> Rate Limiter Dynamic/2
  Constant2/1 -> Rate Limiter Dynamic/1
  Constant3/1 -> Rate Limiter Dynamic/3

== system Inverter2016a/3ph- Module1/Gate Driver1/Voltage Measure3 ==
  PS-Simulink Converter2 : nesl_utility/PS-Simulink Converter  PhysicalDomain=network_engine_domain  SubClassName=ps_output  LeftPortType=input  RightPortType=output  PseudoPeriodic=off  Frequencies=[]  Unit=1  AffineConversion=off
  Voltage Sensor3 : fl_lib/Electrical/Electrical Sensors/Voltage Sensor
  V+ : PMIOPort  Side=Right
  V- : PMIOPort  Port=2  Side=Right
  Data : Outport
  wires:
  PS-Simulink Converter2/1 -> Data/1
  connections:
  PS-Simulink Converter2/LConn1 -- Voltage Sensor3/RConn1
  Voltage Sensor3/RConn2 -- V-/RConn1
  Voltage Sensor3/LConn1 -- V+/RConn1

== system Inverter2016a/3ph- Module1/Gate Driver2/Current Measure ==
  Current Sensor1 : fl_lib/Electrical/Electrical Sensors/Current Sensor
  PS-Simulink Converter4 : nesl_utility/PS-Simulink Converter  PhysicalDomain=network_engine_domain  SubClassName=ps_output  LeftPortType=input  RightPortType=output  PseudoPeriodic=off  Frequencies=[]  Unit=1  AffineConversion=off
  I+ : PMIOPort  Side=Left
  I- : PMIOPort  Port=2  Side=Right
  Data : Outport
  wires:
  PS-Simulink Converter4/1 -> Data/1
  connections:
  Current Sensor1/LConn1 -- I+/RConn1
  PS-Simulink Converter4/LConn1 -- Current Sensor1/RConn1
  Current Sensor1/RConn2 -- I-/RConn1

== system Inverter2016a/3ph- Module1/Gate Driver2/Rate Limiter2 ==
  Inp : Inport
  Constant2 : Constant  Value=(VpulseMax - VpulseMin)/1e-9
  Constant3 : Constant  Value=(VpulseMin - VpulseMax)/1e-9
  Rate Limiter Dynamic : simulink/Discontinuities/Rate Limiter Dynamic
  Outp : Outport
  wires:
  Rate Limiter Dynamic/1 -> Outp/1
  Inp/1 -> Rate Limiter Dynamic/2
  Constant2/1 -> Rate Limiter Dynamic/1
  Constant3/1 -> Rate Limiter Dynamic/3

== system Inverter2016a/3ph- Module1/Gate Driver2/Voltage Measure3 ==
  PS-Simulink Converter2 : nesl_utility/PS-Simulink Converter  PhysicalDomain=network_engine_domain  SubClassName=ps_output  LeftPortType=input  RightPortType=output  PseudoPeriodic=off  Frequencies=[]  Unit=1  AffineConversion=off
  Voltage Sensor3 : fl_lib/Electrical/Electrical Sensors/Voltage Sensor
  V+ : PMIOPort  Side=Right
  V- : PMIOPort  Port=2  Side=Right
  Data : Outport
  wires:
  PS-Simulink Converter2/1 -> Data/1
  connections:
  PS-Simulink Converter2/LConn1 -- Voltage Sensor3/RConn1
  Voltage Sensor3/RConn2 -- V-/RConn1
  Voltage Sensor3/LConn1 -- V+/RConn1

== system Inverter2016a/3ph- Module1/Gate Driver3/Current Measure ==
  Current Sensor1 : fl_lib/Electrical/Electrical Sensors/Current Sensor
  PS-Simulink Converter4 : nesl_utility/PS-Simulink Converter  PhysicalDomain=network_engine_domain  SubClassName=ps_output  LeftPortType=input  RightPortType=output  PseudoPeriodic=off  Frequencies=[]  Unit=1  AffineConversion=off
  I+ : PMIOPort  Side=Left
  I- : PMIOPort  Port=2  Side=Right
  Data : Outport
  wires:
  PS-Simulink Converter4/1 -> Data/1
  connections:
  Current Sensor1/LConn1 -- I+/RConn1
  PS-Simulink Converter4/LConn1 -- Current Sensor1/RConn1
  Current Sensor1/RConn2 -- I-/RConn1

== system Inverter2016a/3ph- Module1/Gate Driver3/Rate Limiter2 ==
  Inp : Inport
  Constant2 : Constant  Value=(VpulseMax - VpulseMin)/1e-9
  Constant3 : Constant  Value=(VpulseMin - VpulseMax)/1e-9
  Rate Limiter Dynamic : simulink/Discontinuities/Rate Limiter Dynamic
  Outp : Outport
  wires:
  Rate Limiter Dynamic/1 -> Outp/1
  Inp/1 -> Rate Limiter Dynamic/2
  Constant2/1 -> Rate Limiter Dynamic/1
  Constant3/1 -> Rate Limiter Dynamic/3

== system Inverter2016a/3ph- Module1/Gate Driver3/Voltage Measure3 ==
  PS-Simulink Converter2 : nesl_utility/PS-Simulink Converter  PhysicalDomain=network_engine_domain  SubClassName=ps_output  LeftPortType=input  RightPortType=output  PseudoPeriodic=off  Frequencies=[]  Unit=1  AffineConversion=off
  Voltage Sensor3 : fl_lib/Electrical/Electrical Sensors/Voltage Sensor
  V+ : PMIOPort  Side=Right
  V- : PMIOPort  Port=2  Side=Right
  Data : Outport
  wires:
  PS-Simulink Converter2/1 -> Data/1
  connections:
  PS-Simulink Converter2/LConn1 -- Voltage Sensor3/RConn1
  Voltage Sensor3/RConn2 -- V-/RConn1
  Voltage Sensor3/LConn1 -- V+/RConn1

== system Inverter2016a/3ph- Module1/Gate Driver4/Current Measure ==
  Current Sensor1 : fl_lib/Electrical/Electrical Sensors/Current Sensor
  PS-Simulink Converter4 : nesl_utility/PS-Simulink Converter  PhysicalDomain=network_engine_domain  SubClassName=ps_output  LeftPortType=input  RightPortType=output  PseudoPeriodic=off  Frequencies=[]  Unit=1  AffineConversion=off
  I+ : PMIOPort  Side=Left
  I- : PMIOPort  Port=2  Side=Right
  Data : Outport
  wires:
  PS-Simulink Converter4/1 -> Data/1
  connections:
  Current Sensor1/LConn1 -- I+/RConn1
  PS-Simulink Converter4/LConn1 -- Current Sensor1/RConn1
  Current Sensor1/RConn2 -- I-/RConn1

== system Inverter2016a/3ph- Module1/Gate Driver4/Rate Limiter2 ==
  Inp : Inport
  Constant2 : Constant  Value=(VpulseMax - VpulseMin)/1e-9
  Constant3 : Constant  Value=(VpulseMin - VpulseMax)/1e-9
  Rate Limiter Dynamic : simulink/Discontinuities/Rate Limiter Dynamic
  Outp : Outport
  wires:
  Rate Limiter Dynamic/1 -> Outp/1
  Inp/1 -> Rate Limiter Dynamic/2
  Constant2/1 -> Rate Limiter Dynamic/1
  Constant3/1 -> Rate Limiter Dynamic/3

== system Inverter2016a/3ph- Module1/Gate Driver4/Voltage Measure3 ==
  PS-Simulink Converter2 : nesl_utility/PS-Simulink Converter  PhysicalDomain=network_engine_domain  SubClassName=ps_output  LeftPortType=input  RightPortType=output  PseudoPeriodic=off  Frequencies=[]  Unit=1  AffineConversion=off
  Voltage Sensor3 : fl_lib/Electrical/Electrical Sensors/Voltage Sensor
  V+ : PMIOPort  Side=Right
  V- : PMIOPort  Port=2  Side=Right
  Data : Outport
  wires:
  PS-Simulink Converter2/1 -> Data/1
  connections:
  PS-Simulink Converter2/LConn1 -- Voltage Sensor3/RConn1
  Voltage Sensor3/RConn2 -- V-/RConn1
  Voltage Sensor3/LConn1 -- V+/RConn1

== system Inverter2016a/3ph- Module1/Gate Driver5/Current Measure ==
  Current Sensor1 : fl_lib/Electrical/Electrical Sensors/Current Sensor
  PS-Simulink Converter4 : nesl_utility/PS-Simulink Converter  PhysicalDomain=network_engine_domain  SubClassName=ps_output  LeftPortType=input  RightPortType=output  PseudoPeriodic=off  Frequencies=[]  Unit=1  AffineConversion=off
  I+ : PMIOPort  Side=Left
  I- : PMIOPort  Port=2  Side=Right
  Data : Outport
  wires:
  PS-Simulink Converter4/1 -> Data/1
  connections:
  Current Sensor1/LConn1 -- I+/RConn1
  PS-Simulink Converter4/LConn1 -- Current Sensor1/RConn1
  Current Sensor1/RConn2 -- I-/RConn1

== system Inverter2016a/3ph- Module1/Gate Driver5/Rate Limiter2 ==
  Inp : Inport
  Constant2 : Constant  Value=(VpulseMax - VpulseMin)/1e-9
  Constant3 : Constant  Value=(VpulseMin - VpulseMax)/1e-9
  Rate Limiter Dynamic : simulink/Discontinuities/Rate Limiter Dynamic
  Outp : Outport
  wires:
  Rate Limiter Dynamic/1 -> Outp/1
  Inp/1 -> Rate Limiter Dynamic/2
  Constant2/1 -> Rate Limiter Dynamic/1
  Constant3/1 -> Rate Limiter Dynamic/3

== system Inverter2016a/3ph- Module1/Gate Driver5/Voltage Measure3 ==
  PS-Simulink Converter2 : nesl_utility/PS-Simulink Converter  PhysicalDomain=network_engine_domain  SubClassName=ps_output  LeftPortType=input  RightPortType=output  PseudoPeriodic=off  Frequencies=[]  Unit=1  AffineConversion=off
  Voltage Sensor3 : fl_lib/Electrical/Electrical Sensors/Voltage Sensor
  V+ : PMIOPort  Side=Right
  V- : PMIOPort  Port=2  Side=Right
  Data : Outport
  wires:
  PS-Simulink Converter2/1 -> Data/1
  connections:
  PS-Simulink Converter2/LConn1 -- Voltage Sensor3/RConn1
  Voltage Sensor3/RConn2 -- V-/RConn1
  Voltage Sensor3/LConn1 -- V+/RConn1

== system Inverter2016a/3ph- Module1/R L Load/Current Measure1 ==
  Current Sensor1 : fl_lib/Electrical/Electrical Sensors/Current Sensor
  PS-Simulink Converter4 : nesl_utility/PS-Simulink Converter  PhysicalDomain=network_engine_domain  SubClassName=ps_output  LeftPortType=input  RightPortType=output  PseudoPeriodic=off  Frequencies=[]  Unit=1  AffineConversion=off
  I+ : PMIOPort  Side=Left
  I- : PMIOPort  Port=2  Side=Right
  Data : Outport
  wires:
  PS-Simulink Converter4/1 -> Data/1
  connections:
  Current Sensor1/RConn2 -- I-/RConn1
  PS-Simulink Converter4/LConn1 -- Current Sensor1/RConn1
  Current Sensor1/LConn1 -- I+/RConn1

== system Inverter2016a/3ph- Module1/R L Load/Current Measure2 ==
  Current Sensor1 : fl_lib/Electrical/Electrical Sensors/Current Sensor
  PS-Simulink Converter4 : nesl_utility/PS-Simulink Converter  PhysicalDomain=network_engine_domain  SubClassName=ps_output  LeftPortType=input  RightPortType=output  PseudoPeriodic=off  Frequencies=[]  Unit=1  AffineConversion=off
  I+ : PMIOPort  Side=Left
  I- : PMIOPort  Port=2  Side=Right
  Data : Outport
  wires:
  PS-Simulink Converter4/1 -> Data/1
  connections:
  Current Sensor1/LConn1 -- I+/RConn1
  PS-Simulink Converter4/LConn1 -- Current Sensor1/RConn1
  Current Sensor1/RConn2 -- I-/RConn1

== system Inverter2016a/3ph- Module1/R L Load/Current Measure5 ==
  Current Sensor1 : fl_lib/Electrical/Electrical Sensors/Current Sensor
  PS-Simulink Converter4 : nesl_utility/PS-Simulink Converter  PhysicalDomain=network_engine_domain  SubClassName=ps_output  LeftPortType=input  RightPortType=output  PseudoPeriodic=off  Frequencies=[]  Unit=1  AffineConversion=off
  I+ : PMIOPort  Side=Left
  I- : PMIOPort  Port=2  Side=Right
  Data : Outport
  wires:
  PS-Simulink Converter4/1 -> Data/1
  connections:
  Current Sensor1/LConn1 -- I+/RConn1
  PS-Simulink Converter4/LConn1 -- Current Sensor1/RConn1
  Current Sensor1/RConn2 -- I-/RConn1

== system Inverter2016a/3ph- Module1/R L Load/Voltage Measure1 ==
  PS-Simulink Converter2 : nesl_utility/PS-Simulink Converter  PhysicalDomain=network_engine_domain  SubClassName=ps_output  LeftPortType=input  RightPortType=output  PseudoPeriodic=off  Frequencies=[]  Unit=1  AffineConversion=off
  Voltage Sensor3 : fl_lib/Electrical/Electrical Sensors/Voltage Sensor
  V+ : PMIOPort  Side=Right
  V- : PMIOPort  Port=2  Side=Right
  Data : Outport
  wires:
  PS-Simulink Converter2/1 -> Data/1
  connections:
  Voltage Sensor3/LConn1 -- V+/RConn1
  Voltage Sensor3/RConn2 -- V-/RConn1
  PS-Simulink Converter2/LConn1 -- Voltage Sensor3/RConn1

== system Inverter2016a/3ph- Module1/R L Load/Voltage Measure2 ==
  PS-Simulink Converter2 : nesl_utility/PS-Simulink Converter  PhysicalDomain=network_engine_domain  SubClassName=ps_output  LeftPortType=input  RightPortType=output  PseudoPeriodic=off  Frequencies=[]  Unit=1  AffineConversion=off
  Voltage Sensor3 : fl_lib/Electrical/Electrical Sensors/Voltage Sensor
  V+ : PMIOPort  Side=Right
  V- : PMIOPort  Port=2  Side=Right
  Data : Outport
  wires:
  PS-Simulink Converter2/1 -> Data/1
  connections:
  PS-Simulink Converter2/LConn1 -- Voltage Sensor3/RConn1
  Voltage Sensor3/RConn2 -- V-/RConn1
  Voltage Sensor3/LConn1 -- V+/RConn1

== system Inverter2016a/3ph- Module1/R L Load/Voltage Measure3 ==
  PS-Simulink Converter2 : nesl_utility/PS-Simulink Converter  PhysicalDomain=network_engine_domain  SubClassName=ps_output  LeftPortType=input  RightPortType=output  PseudoPeriodic=off  Frequencies=[]  Unit=1  AffineConversion=off
  Voltage Sensor3 : fl_lib/Electrical/Electrical Sensors/Voltage Sensor
  V+ : PMIOPort  Side=Right
  V- : PMIOPort  Port=2  Side=Right
  Data : Outport
  wires:
  PS-Simulink Converter2/1 -> Data/1
  connections:
  PS-Simulink Converter2/LConn1 -- Voltage Sensor3/RConn1
  Voltage Sensor3/RConn2 -- V-/RConn1
  Voltage Sensor3/LConn1 -- V+/RConn1
